simulink model "chap10_7sim"  (Simulink 3.00)
settings: Solver=ode45  StartTime=0.0  StopTime=3  FixedStep=0.001  RelTol=1e-3
settings Model: LastModifiedBy=liu

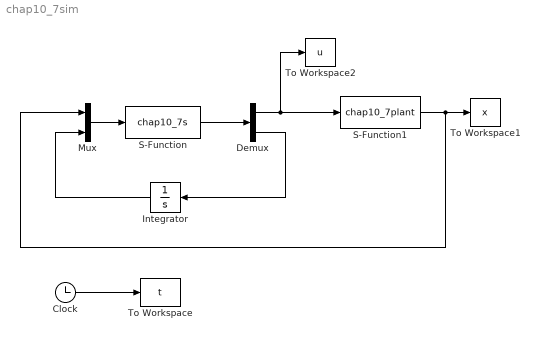
== system chap10_7sim ==
  Clock : Clock
      settings: DisplayTime=off  Decimation=10
  Demux : Demux  Outputs=2
  Integrator : Integrator  Orientation=left  ExternalReset=none  InitialConditionSource=internal  InitialCondition=0  LimitOutput=off  UpperSaturationLimit=inf  LowerSaturationLimit=-inf  ShowSaturationPort=off  ShowStatePort=off  AbsoluteTolerance=auto
  Mux : Mux  Inputs=2
  S-Function : S-Function  FunctionName=chap10_7s  PortCounts=[]  SFunctionModules=''
  S-Function1 : S-Function  FunctionName=chap10_7plant  PortCounts=[]  SFunctionModules=''
  To Workspace : ToWorkspace  VariableName=t  SampleTime=-1  SaveFormat=Matrix
  To Workspace1 : ToWorkspace  VariableName=x  SampleTime=-1  SaveFormat=Matrix
  To Workspace2 : ToWorkspace  VariableName=u  SampleTime=-1  SaveFormat=Matrix
  wires:
  Clock/1 -> To Workspace/1
  S-Function/1 -> Demux/1
  Demux/1 -> S-Function1/1, To Workspace2/1
  Demux/2 -> Integrator/1
  Mux/1 -> S-Function/1
  Integrator/1 -> Mux/2
  S-Function1/1 -> To Workspace1/1, Mux/1
